simulink model "adaptive_observer_for_sin_signal_original"  (R2021b)
settings: Solver=ode4  StartTime=0.0  StopTime=200.0  FixedStep=0.0001  RelTol=1e-3
model workspace: external: MATLAB File D:\practice\sci\variables2n1.m (data not in the file)
values from neighbouring files (symbols this model uses):
  A = zeros(2*dimension+1 , 2*dimension+1)    [variables2n1.m]
  alpha = [1,3]    [variables2n1.m]
  amp = [1;1]    [variables2n1.m]
  amp_M = [1;1]    [variables2n1.m]
  bias = [0;0]    [variables2n1.m]
  bias_M = [0;0]    [variables2n1.m]
  bigGammaZ0 = zeros(2*dimension+1, dimension)    [variables2n1.m]
  C = zeros(1, 2*dimension+1)    [variables2n1.m]
  delta = C*A    [variables2n1.m]
  dimension = 2    [variables2n1.m]
  freq = [2;3]    [variables2n1.m]
  freq_M = [1.8;3.2]    [variables2n1.m]
  freqSwitcher = 100    [variables2n1.m]
  initialTheta = [initialOmega(1)^2-alpha(1);     initialOmega(2)^2-alpha(2)]    [variables2n1.m]
  initialZ = [1*sin(0); 1*r^2*cos(0)/initialOmega(1);           1*sin(0); 1*r^2*cos(0)/initialOmega(2); 0]    [variables2n1.m]
  L = (place(A',C',eigenvalues))'    [variables2n1.m]
  mu = 2    [variables2n1.m]
  omegaLimiter = sqrt(dimension)*maxOmega    [variables2n1.m]
  phase = [0;0]    [variables2n1.m]
  phase_M = [0;0]    [variables2n1.m]
  r = 1.2    [variables2n1.m]
  turn_mods_on = 0    [variables2n1.m]
  zMax = 5    [variables2n1.m]
undefined symbols (not defined in the file or in its folder): G
settings Model: Creator=ASUS  LastModifiedBy=ASUS

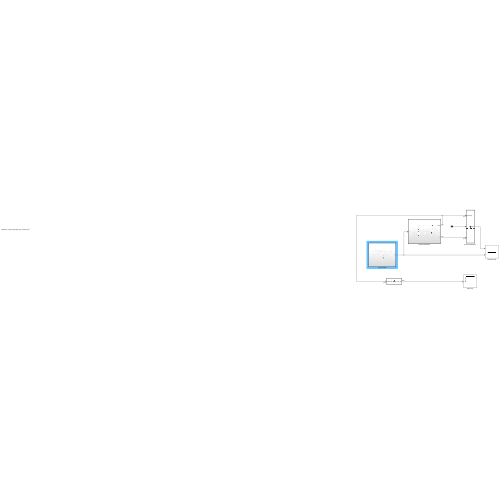
[thumbnail: Simulink's stored preview of the top-level diagram]
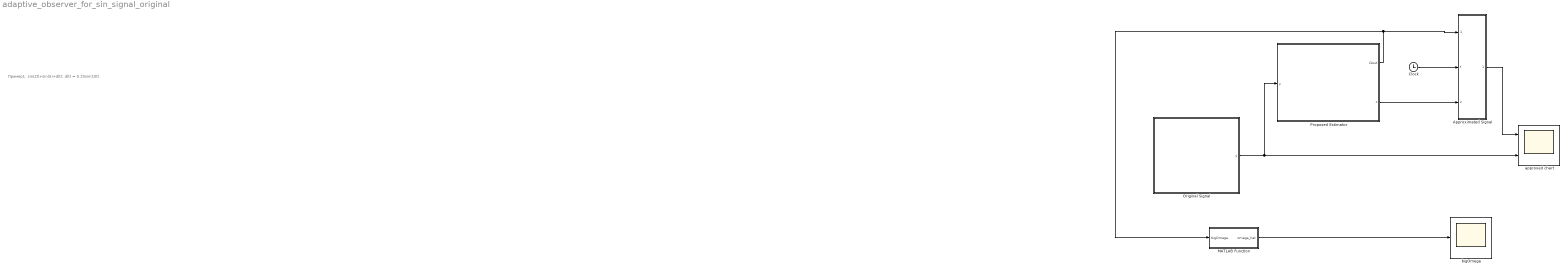
== system adaptive_observer_for_sin_signal_original ==
  note: Пример1. sin(2t)+sin(5)+d(t); d(t) = 0.25sin(10t)
  Approximated Signal : MATLAB Function  TreatAsAtomicUnit=on
  Clock : Clock
  MATLAB Function : MATLAB Function  TreatAsAtomicUnit=on
  Original Signal : Subsystem  Priority=1  TreatAsAtomicUnit=on
  Proposed Estimator : Subsystem  Priority=2  TreatAsAtomicUnit=on
  approxed chart : Scope  NumInputPorts=2
  bigOmega : Scope
  wires:
  Approximated Signal/1(sgn_value) -> approxed chart/1
  Clock/1 -> Approximated Signal/2(t)
  Original Signal/1(y) -> approxed chart/2, Proposed Estimator/1(y)
  Proposed Estimator/2(z) -> Approximated Signal/3(z)
  Proposed Estimator/1(Ωout) -> Approximated Signal/1(bigOmega), MATLAB Function/1(bigOmega)
  MATLAB Function/1(omega_hat) -> bigOmega/1

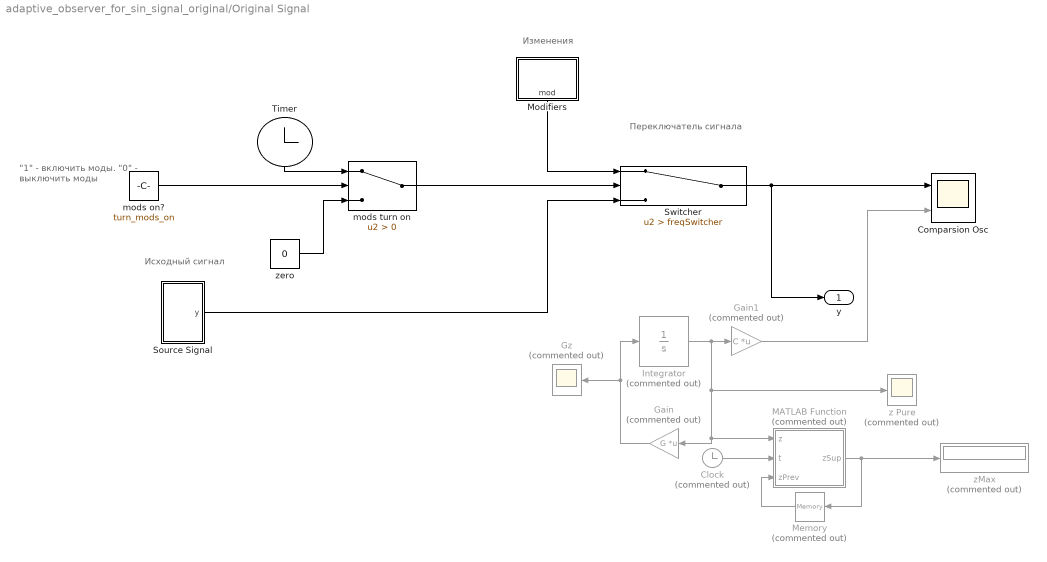
== system adaptive_observer_for_sin_signal_original/Original Signal ==
  note: "1" - включить моды.
      | "0" - выключить моды
  note: Изменения
  note: Переключатель сигнала
  note: Исходный сигнал
  Clock : Clock  Commented=on
  Comparsion Osc : Scope  NumInputPorts=2
  Gain : Gain  Commented=on  Gain=G  Multiplication=Matrix(K*u)
  Gain1 : Gain  Commented=on  Gain=C  Multiplication=Matrix(K*u)
  Gz : Scope  Commented=on
  Integrator : Integrator  Commented=on  InitialCondition=[0;(r^2)/2;0;(r^2)/3;0]
  MATLAB Function : MATLAB Function  Commented=on  TreatAsAtomicUnit=on
  Memory : Memory  Commented=on
  Modifiers : Subsystem
  Source Signal : Subsystem
  Switcher : Switch  Criteria=u2 > Threshold  Threshold=freqSwitcher
  Timer : Clock
  mods on? : Constant  Value=turn_mods_on
  mods turn on : Switch  Criteria=u2 > Threshold
  z Pure : Scope  Commented=on
  zMax : Display  Commented=on
  zero : Constant  Value=0
  y : Outport
  wires:
  Gain/1 -> Gz/1, Integrator/1
  Gain1/1 -> Comparsion Osc/2
  Integrator/1 -> Gain/1, MATLAB Function/1(z), z Pure/1, Gain1/1
  MATLAB Function/1(zSup) -> Memory/1, zMax/1
  Clock/1 -> MATLAB Function/2(t)
  Memory/1 -> MATLAB Function/3(zPrev)
  Source Signal/1(y) -> Switcher/3
  Modifiers/1(mod) -> Switcher/1
  Switcher/1 -> y/1, Comparsion Osc/1
  mods on?/1 -> mods turn on/2
  Timer/1 -> mods turn on/1
  mods turn on/1 -> Switcher/2
  zero/1 -> mods turn on/3

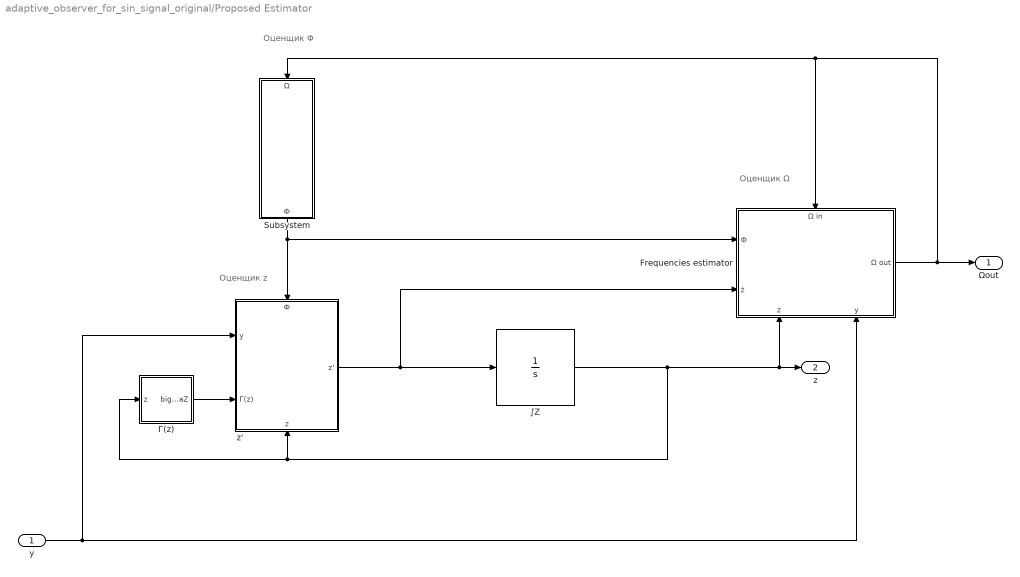
== system adaptive_observer_for_sin_signal_original/Proposed Estimator ==
  note: Оценщик Ω
  note: Оценщик Φ
  note: Оценщик z
  y : Inport
  Frequencies estimator : Subsystem
      settings: PortSchema="{\"entries\":[{\"content\":{\"sides\":[{\"content\":{\"connectorIds\":[\"In1\",\"In2\"]},\"type\":\"ConnectorPlacement.EquallySpacedRectSide\",\"uuid\":\"56415c13-d553-4f88-94d3-75bcdc800e4b\"},{\"content\":{\"connectorIds\":[\"Out1\"],\"side\":\"RIGHT\"},\"type\":\"ConnectorPlacement.EquallySpacedRectSide\",\"uuid\":\"a1bdd2d2-4e49-40cb-b0b7-1df5316e4510\"},{\"content\":{\"connectorIds\":[\"In3\"],\"side\":\"TOP\"},\"type\":\"ConnectorPlacement.EquallySpacedRectSide\",\"uuid\":\"59b6ba3d-4a55-43e8-9b14-0d873cc3c9ca\"},{\"content\":{\"connectorIds\":[\"In4\",\"In5\"],\"side\":\"BOTTOM\"},\"type\":\"ConnectorPlacement.EquallySpacedRectSide\",\"uuid\":\"70a04625-4f15-4458-8acb-2ccaa963f28c\"}]},\"type\":\"ConnectorPlacement.EquallySpacedConnector\",\"uuid\":\"fdf2e112-ecff-41aa-a5cb-d527a9dd51a8\"}],\"packageUris\":[\"http://schema.mathworks.com/mf0/Connector/R2020b\"],\"version\":\"1.0\"}"
  Subsystem : Subsystem  Priority=6  TreatAsAtomicUnit=on
  z' : Subsystem  Priority=7  TreatAsAtomicUnit=on
      settings: PortSchema="{\"entries\":[{\"content\":{\"sides\":[{\"content\":{\"connectorIds\":[\"In1\",\"In2\"]},\"type\":\"ConnectorPlacement.EquallySpacedRectSide\",\"uuid\":\"ef8cffdc-1e6f-42c0-8cb3-bf318ca182f8\"},{\"content\":{\"connectorIds\":[\"Out1\"],\"side\":\"RIGHT\"},\"type\":\"ConnectorPlacement.EquallySpacedRectSide\",\"uuid\":\"a9c7e5b7-281a-47aa-808a-eb2877f3eee0\"},{\"content\":{\"connectorIds\":[\"In3\"],\"side\":\"TOP\"},\"type\":\"ConnectorPlacement.EquallySpacedRectSide\",\"uuid\":\"7bb4f6b5-7deb-4e08-9b2d-b96cfbb2c85e\"},{\"content\":{\"connectorIds\":[\"In4\"],\"side\":\"BOTTOM\"},\"type\":\"ConnectorPlacement.EquallySpacedRectSide\",\"uuid\":\"fa3b2d15-5a15-4cf8-893e-51642802107c\"}]},\"type\":\"ConnectorPlacement.EquallySpacedConnector\",\"uuid\":\"64fccc24-315d-40ff-920f-bd434d551c1a\"}],\"packageUris\":[\"http://schema.mathworks.com/mf0/Connector/R2020b\"],\"version\":\"1.0\"}"
  Г(z) : MATLAB Function  Priority=2  TreatAsAtomicUnit=on
  "∫Z " : Integrator  Priority=1  InitialCondition=initialZ
  Ωout : Outport
  z : Outport  Port=2
  wires:
  z'/1(z') -> Frequencies estimator/2(ż), "∫Z "/1
  Г(z)/1(bigGammaZ) -> z'/2(Г(z))
  "∫Z "/1 -> z/1, Frequencies estimator/4(z), Г(z)/1(z), z'/4(z)
  Frequencies estimator/1(Ω out) -> Subsystem/1(Ω), Frequencies estimator/3(Ω in), Ωout/1
  y/1 -> Frequencies estimator/5(y), z'/1(y)
  Subsystem/1(Ф) -> z'/3(Ф), Frequencies estimator/1(Ф)

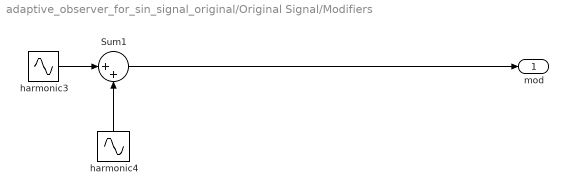
== system adaptive_observer_for_sin_signal_original/Original Signal/Modifiers ==
  Sum1 : Sum  Inputs=|++
  harmonic3 : Sin  Priority=0  Amplitude=amp_M(1)  Bias=bias_M(1)  Frequency=freq_M(1)  Phase=phase_M(1)  SampleTime=0
  harmonic4 : Sin  Priority=0  Amplitude=amp_M(2)  Bias=bias_M(2)  Frequency=freq_M(2)  Phase=phase_M(2)  SampleTime=0
  mod : Outport
  wires:
  harmonic4/1 -> Sum1/2
  harmonic3/1 -> Sum1/1
  Sum1/1 -> mod/1

== system adaptive_observer_for_sin_signal_original/Original Signal/Source Signal ==
  Sum : Sum  Inputs=|++
  harmonic1 : Sin  Priority=0  Amplitude=amp(1)  Bias=bias(1)  Frequency=freq(1)  Phase=phase(1)  SampleTime=0
  harmonic2 : Sin  Priority=0  Amplitude=amp(2)  Bias=bias(2)  Frequency=freq(2)  Phase=phase(2)  SampleTime=0
  y : Outport
  wires:
  harmonic1/1 -> Sum/1
  harmonic2/1 -> Sum/2
  Sum/1 -> y/1

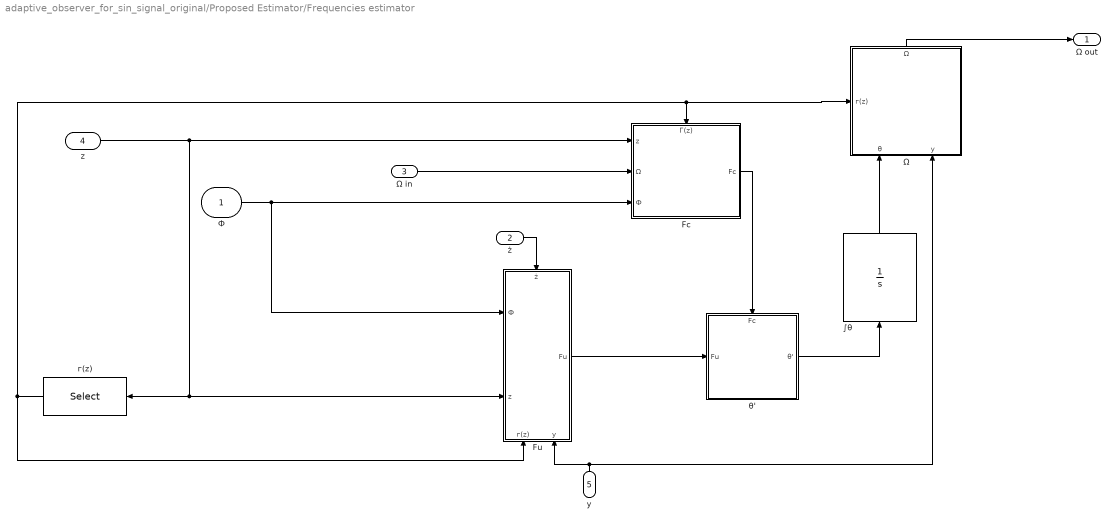
== system adaptive_observer_for_sin_signal_original/Proposed Estimator/Frequencies estimator ==
  Ф : Inport
  ż : Inport  Port=2
  Ω in : Inport  Port=3
  z : Inport  Port=4
  y : Inport  Port=5
  Fc : Subsystem  Priority=8  TreatAsAtomicUnit=on
      settings: PortSchema="{\"entries\":[{\"content\":{\"sides\":[{\"content\":{\"connectorIds\":[\"In1\",\"In2\",\"In3\"]},\"type\":\"ConnectorPlacement.EquallySpacedRectSide\",\"uuid\":\"ef8cffdc-1e6f-42c0-8cb3-bf318ca182f8\"},{\"content\":{\"connectorIds\":[\"Out1\"],\"side\":\"RIGHT\"},\"type\":\"ConnectorPlacement.EquallySpacedRectSide\",\"uuid\":\"a9c7e5b7-281a-47aa-808a-eb2877f3eee0\"},{\"content\":{\"connectorIds\":[\"In4\"],\"side\":\"TOP\"},\"type\":\"ConnectorPlacement.EquallySpacedRectSide\",\"uuid\":\"7bb4f6b5-7deb-4e08-9b2d-b96cfbb2c85e\"},{\"content\":{\"connectorIds\":[],\"side\":\"BOTTOM\"},\"type\":\"ConnectorPlacement.EquallySpacedRectSide\",\"uuid\":\"d628d464-6f95-4c60-8de5-a9188665a8a2\"}]},\"type\":\"ConnectorPlacement.EquallySpacedConnector\",\"uuid\":\"64fccc24-315d-40ff-920f-bd434d551c1a\"}],\"packageUris\":[\"http://schema.mathworks.com/mf0/Connector/R2020b\"],\"version\":\"1.0\"}"
  Fu : Subsystem  Priority=9  TreatAsAtomicUnit=on
      settings: PortSchema="{\"entries\":[{\"content\":{\"sides\":[{\"content\":{\"connectorIds\":[\"In1\",\"In2\"]},\"type\":\"ConnectorPlacement.EquallySpacedRectSide\",\"uuid\":\"56415c13-d553-4f88-94d3-75bcdc800e4b\"},{\"content\":{\"connectorIds\":[\"Out1\"],\"side\":\"RIGHT\"},\"type\":\"ConnectorPlacement.EquallySpacedRectSide\",\"uuid\":\"a1bdd2d2-4e49-40cb-b0b7-1df5316e4510\"},{\"content\":{\"connectorIds\":[\"In3\"],\"side\":\"TOP\"},\"type\":\"ConnectorPlacement.EquallySpacedRectSide\",\"uuid\":\"59b6ba3d-4a55-43e8-9b14-0d873cc3c9ca\"},{\"content\":{\"connectorIds\":[\"In4\",\"In5\"],\"side\":\"BOTTOM\"},\"type\":\"ConnectorPlacement.EquallySpacedRectSide\",\"uuid\":\"cb3db39e-f643-4fe7-a27f-76e86359c78d\"}]},\"type\":\"ConnectorPlacement.EquallySpacedConnector\",\"uuid\":\"fdf2e112-ecff-41aa-a5cb-d527a9dd51a8\"}],\"packageUris\":[\"http://schema.mathworks.com/mf0/Connector/R2020b\"],\"version\":\"1.0\"}"
  Ω : Subsystem  Priority=5  TreatAsAtomicUnit=on
      settings: PortSchema="{\"entries\":[{\"content\":{\"sides\":[{\"content\":{\"connectorIds\":[\"In1\",\"In2\"]},\"type\":\"ConnectorPlacement.EquallySpacedRectSide\",\"uuid\":\"0172ca52-64e8-432c-895c-e5829558e278\"},{\"content\":{\"connectorIds\":[\"Out1\"],\"side\":\"RIGHT\"},\"type\":\"ConnectorPlacement.EquallySpacedRectSide\",\"uuid\":\"c83f4e01-5d94-498a-a9de-b4a302d500ab\"},{\"content\":{\"connectorIds\":[\"In3\"],\"side\":\"TOP\"},\"type\":\"ConnectorPlacement.EquallySpacedRectSide\",\"uuid\":\"3a6496e3-470c-4361-9f8f-cd28e1556398\"}]},\"type\":\"ConnectorPlacement.EquallySpacedConnector\",\"uuid\":\"b738ec8a-20ee-4a0a-8362-4988f331d970\"}],\"packageUris\":[\"http://schema.mathworks.com/mf0/Connector/R2020b\"],\"version\":\"1.0\"}"
  θ' : Subsystem  Priority=10  TreatAsAtomicUnit=on
      settings: PortSchema="{\"entries\":[{\"content\":{\"sides\":[{\"content\":{\"connectorIds\":[\"In1\"]},\"type\":\"ConnectorPlacement.EquallySpacedRectSide\",\"uuid\":\"9184f415-d771-478b-8114-38f854f6aad6\"},{\"content\":{\"connectorIds\":[\"Out1\"],\"side\":\"RIGHT\"},\"type\":\"ConnectorPlacement.EquallySpacedRectSide\",\"uuid\":\"399c2935-e635-4d1c-9ba7-451eea57bae3\"},{\"content\":{\"connectorIds\":[\"In2\"],\"side\":\"TOP\"},\"type\":\"ConnectorPlacement.EquallySpacedRectSide\",\"uuid\":\"bdc6ec05-8dca-4996-ba70-702aa29fd179\"}]},\"type\":\"ConnectorPlacement.EquallySpacedConnector\",\"uuid\":\"fa68c3f3-8285-4ee8-b99d-908dba81143c\"}],\"packageUris\":[\"http://schema.mathworks.com/mf0/Connector/R2020b\"],\"version\":\"1.0\"}"
  г(z) : Selector  InputPortWidth=2*dimension+1  IndexOptions=Index vector (dialog)  Indices=2:2:2*dimension  OutputSizes=1
  "∫θ " : Integrator  Priority=3  InitialCondition=initialTheta
  Ω out : Outport
  wires:
  Ф/1 -> Fu/1(Ф), Fc/3(Ф)
  y/1 -> Ω/2(y), Fu/5(y)
  z/1 -> г(z)/1, Fu/2(z), Fc/1(z)
  г(z)/1 -> Fc/4(Г(z)), Ω/3(г(z)), Fu/4(г(z))
  Ω in/1 -> Fc/2(Ω)
  ż/1 -> Fu/3(ż)
  "∫θ "/1 -> Ω/1(θ)
  Ω/1(Ω) -> Ω out/1
  Fc/1(Fc) -> θ'/2(Fc)
  Fu/1(Fu) -> θ'/1(Fu)
  θ'/1(θ') -> "∫θ "/1

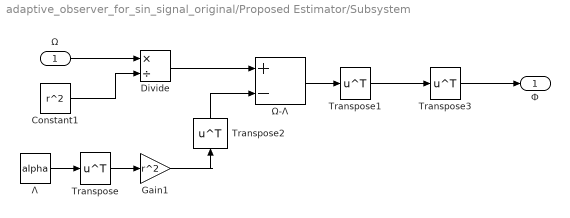
== system adaptive_observer_for_sin_signal_original/Proposed Estimator/Subsystem ==
  Ω : Inport
  Constant1 : Constant  Value=r^2
  Divide : Product  Inputs=*/
  Gain1 : Gain  Gain=r^2
  Transpose{,1..3} (4 alike) : Math  Operator=transpose  SaturateOnIntegerOverflow=on
  Λ : Constant  Value=alpha
  Ω-Λ : Sum  Inputs=+-
  Ф : Outport
  wires:
  Divide/1 -> Ω-Λ/1
  Ω-Λ/1 -> Transpose1/1
  Ω/1 -> Divide/1
  Constant1/1 -> Divide/2
  Gain1/1 -> Transpose2/1
  Λ/1 -> Transpose/1
  Transpose/1 -> Gain1/1
  Transpose2/1 -> Ω-Λ/2
  Transpose1/1 -> Transpose3/1
  Transpose3/1 -> Ф/1

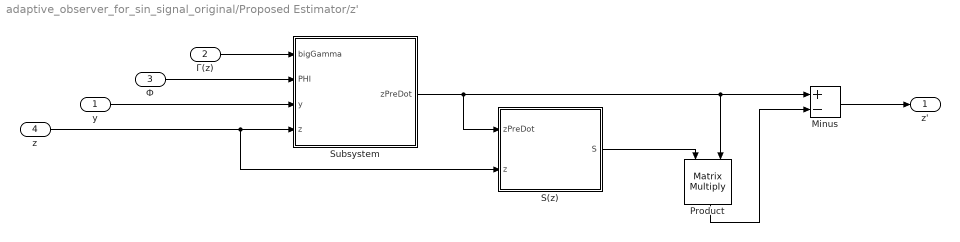
== system adaptive_observer_for_sin_signal_original/Proposed Estimator/z' ==
  y : Inport
  Г(z) : Inport  Port=2
  Ф : Inport  Port=3
  z : Inport  Port=4
  Minus : Sum  Inputs=+-
  Product : Product  Multiplication=Matrix(*)
  S(z) : Subsystem
  Subsystem : Subsystem
  z' : Outport
  wires:
  z/1 -> Subsystem/4(z), S(z)/2(z)
  Minus/1 -> z'/1
  S(z)/1(S) -> Product/1
  Product/1 -> Minus/2
  Subsystem/1(zPreDot) -> Minus/1, Product/2, S(z)/1(zPreDot)
  Г(z)/1 -> Subsystem/1(bigGamma)
  Ф/1 -> Subsystem/2(PHI)
  y/1 -> Subsystem/3(y)

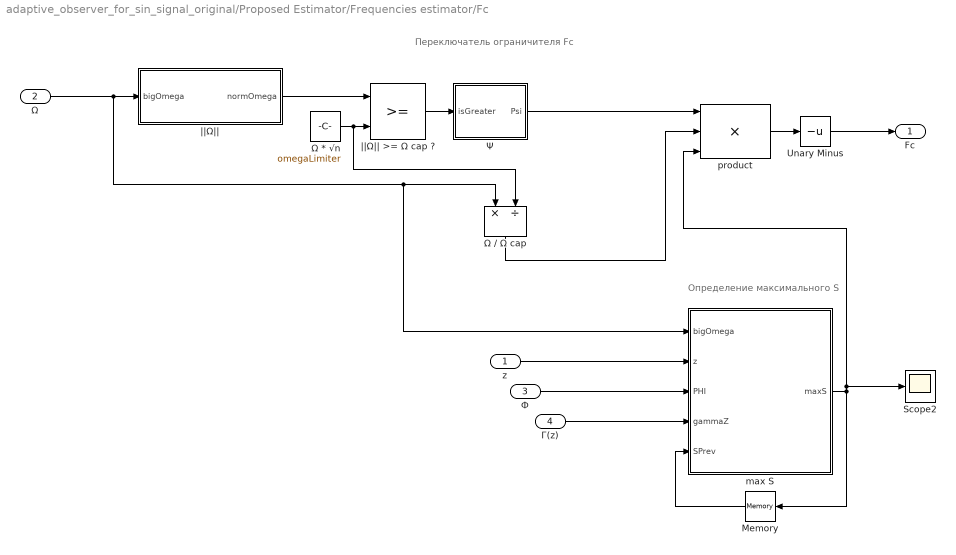
== system adaptive_observer_for_sin_signal_original/Proposed Estimator/Frequencies estimator/Fc ==
  note: Определение максимального S
  note: Переключатель ограничителя Fc
  z : Inport
  Ω : Inport  Port=2
  Ф : Inport  Port=3
  Г(z) : Inport  Port=4
  Memory : Memory
  Scope2 : Scope
  Unary Minus : UnaryMinus
  max S : MATLAB Function  TreatAsAtomicUnit=on
  product : Product  Inputs=3
  ||Ω|| : MATLAB Function  TreatAsAtomicUnit=on
  "||Ω|| >= Ω cap ? " : RelationalOperator  OutDataTypeStr=boolean  RndMeth=Simplest
  Ψ : MATLAB Function  TreatAsAtomicUnit=on
  Ω * √n : Constant  Value=omegaLimiter
  Ω / Ω cap : Product  Inputs=*/
  Fc : Outport
  wires:
  Ф/1 -> max S/3(PHI)
  Ω/1 -> Ω / Ω cap/1, max S/1(bigOmega), ||Ω||/1(bigOmega)
  max S/1(maxS) -> product/3, Scope2/1, Memory/1
  Г(z)/1 -> max S/4(gammaZ)
  z/1 -> max S/2(z)
  ||Ω||/1(normOmega) -> "||Ω|| >= Ω cap ? "/1
  Ω * √n/1 -> Ω / Ω cap/2, "||Ω|| >= Ω cap ? "/2
  "||Ω|| >= Ω cap ? "/1 -> Ψ/1(isGreater)
  Ψ/1(Psi) -> product/1
  Ω / Ω cap/1 -> product/2
  product/1 -> Unary Minus/1
  Unary Minus/1 -> Fc/1
  Memory/1 -> max S/5(SPrev)

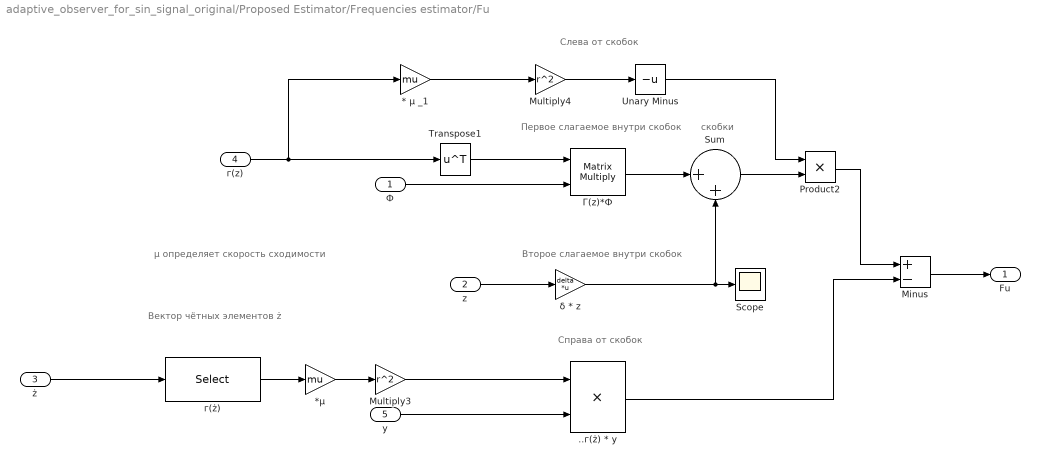
== system adaptive_observer_for_sin_signal_original/Proposed Estimator/Frequencies estimator/Fu ==
  note: Вектор чётных элементов ż
  note: μ определяет скорость сходимости
  note: скобки
  note: Первое слагаемое внутри скобок
  note: Второе слагаемое внутри скобок
  note: Слева от скобок
  note: Справа от скобок
  Ф : Inport
  z : Inport  Port=2
  ż : Inport  Port=3
  г(z) : Inport  Port=4
  y : Inport  Port=5
  * μ _1 : Gain  Gain=mu
  *μ : Gain  Gain=mu
  ..г(ż) * y : Product
  Minus : Sum  Inputs=+-
  Multiply3 : Gain  Gain=r^2
  Multiply4 : Gain  Gain=r^2
  Product2 : Product
  Scope : Scope
  Sum : Sum  Inputs=|++
  Transpose1 : Math  Operator=transpose  SaturateOnIntegerOverflow=on
  Unary Minus : UnaryMinus
  δ * z : Gain  Gain=delta  Multiplication=Matrix(K*u)
  Г(z)*Ф : Product  Multiplication=Matrix(*)
  г(ż) : Selector  InputPortWidth=2*dimension+1  IndexOptions=Index vector (dialog)  Indices=2:2:2*dimension  OutputSizes=1
  Fu : Outport
  wires:
  ż/1 -> г(ż)/1
  г(z)/1 -> * μ _1/1, Transpose1/1
  *μ/1 -> Multiply3/1
  г(ż)/1 -> *μ/1
  Multiply3/1 -> ..г(ż) * y/1
  y/1 -> ..г(ż) * y/2
  Transpose1/1 -> Г(z)*Ф/1
  * μ _1/1 -> Multiply4/1
  Multiply4/1 -> Unary Minus/1
  z/1 -> δ * z/1
  Г(z)*Ф/1 -> Sum/1
  δ * z/1 -> Scope/1, Sum/2
  Unary Minus/1 -> Product2/1
  Sum/1 -> Product2/2
  Product2/1 -> Minus/1
  ..г(ż) * y/1 -> Minus/2
  Minus/1 -> Fu/1
  Ф/1 -> Г(z)*Ф/2

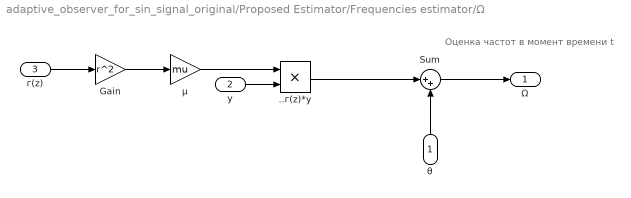
== system adaptive_observer_for_sin_signal_original/Proposed Estimator/Frequencies estimator/Ω ==
  note: Оценка частот в момент времени t
  θ : Inport
  y : Inport  Port=2
  г(z) : Inport  Port=3
  ..г(z)*y : Product
  Gain : Gain  Gain=r^2
  Sum : Sum  Inputs=|++
  μ : Gain  Gain=mu
  Ω : Outport
  wires:
  г(z)/1 -> Gain/1
  Gain/1 -> μ/1
  μ/1 -> ..г(z)*y/1
  y/1 -> ..г(z)*y/2
  ..г(z)*y/1 -> Sum/1
  θ/1 -> Sum/2
  Sum/1 -> Ω/1

== system adaptive_observer_for_sin_signal_original/Proposed Estimator/Frequencies estimator/θ' ==
  note: Образует основу θ'
  note: Удерживает Ω в области определения
  Fu : Inport
  Fc : Inport  Port=2
  Sum : Sum  Inputs=|++
  θ' : Outport
  wires:
  Fu/1 -> Sum/2
  Sum/1 -> θ'/1
  Fc/1 -> Sum/1

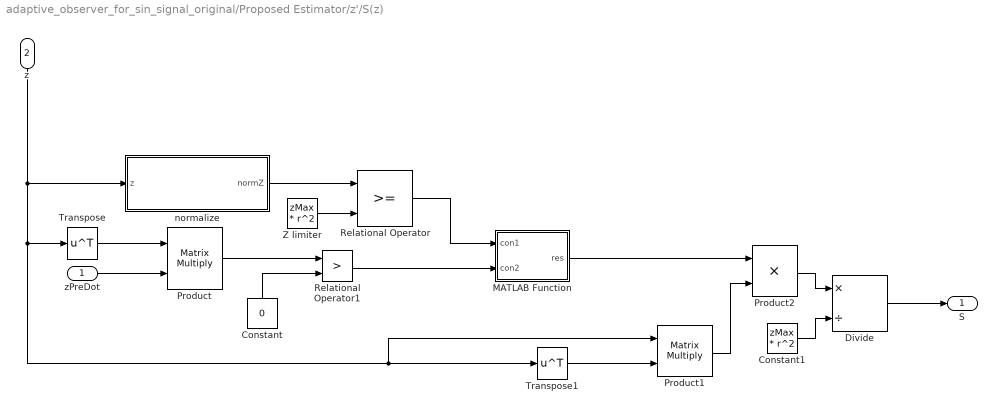
== system adaptive_observer_for_sin_signal_original/Proposed Estimator/z'/S(z) ==
  zPreDot : Inport
  z : Inport  Port=2
  Constant : Constant  Value=0
  Constant1 : Constant  Value=zMax * r^2
  Divide : Product  Inputs=*/
  MATLAB Function : MATLAB Function  TreatAsAtomicUnit=on
  Product : Product  Multiplication=Matrix(*)
  Product1 : Product  Multiplication=Matrix(*)
  Product2 : Product
  Relational Operator : RelationalOperator  OutDataTypeStr=boolean  RndMeth=Simplest
  Relational Operator1 : RelationalOperator  Operator=>  OutDataTypeStr=boolean  RndMeth=Simplest
  Transpose : Math  Operator=transpose  SaturateOnIntegerOverflow=on
  Transpose1 : Math  Operator=transpose  SaturateOnIntegerOverflow=on
  Z limiter : Constant  Value=zMax * r^2
  normalize : MATLAB Function  TreatAsAtomicUnit=on
  S : Outport
  wires:
  Z limiter/1 -> Relational Operator/2
  normalize/1(normZ) -> Relational Operator/1
  Relational Operator/1 -> MATLAB Function/1(con1)
  z/1 -> Product1/1, Transpose1/1, Transpose/1, normalize/1(z)
  Transpose/1 -> Product/1
  zPreDot/1 -> Product/2
  Product/1 -> Relational Operator1/1
  Constant/1 -> Relational Operator1/2
  Relational Operator1/1 -> MATLAB Function/2(con2)
  MATLAB Function/1(res) -> Product2/1
  Transpose1/1 -> Product1/2
  Product1/1 -> Product2/2
  Product2/1 -> Divide/1
  Constant1/1 -> Divide/2
  Divide/1 -> S/1

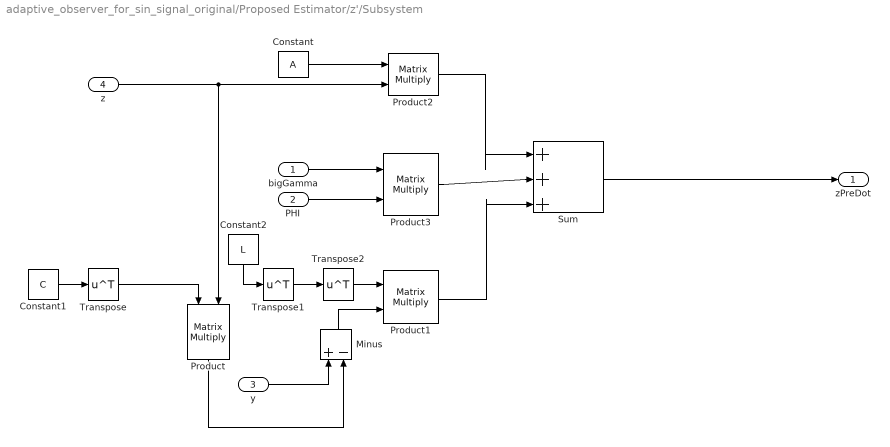
== system adaptive_observer_for_sin_signal_original/Proposed Estimator/z'/Subsystem ==
  bigGamma : Inport
  PHI : Inport  Port=2
  y : Inport  Port=3
  z : Inport  Port=4
  Constant : Constant  Value=A
  Constant1 : Constant  Value=C
  Constant2 : Constant  Value=L
  Minus : Sum  Inputs=+-
  Product{,1..3} (4 alike) : Product  Multiplication=Matrix(*)
  Sum : Sum  Inputs=|+++
  Transpose : Math  Operator=transpose  SaturateOnIntegerOverflow=on
  Transpose1 : Math  Operator=transpose  SaturateOnIntegerOverflow=on
  Transpose2 : Math  Operator=transpose  SaturateOnIntegerOverflow=on
  zPreDot : Outport
  wires:
  z/1 -> Product2/2, Product/2
  Sum/1 -> zPreDot/1
  Constant1/1 -> Transpose/1
  y/1 -> Minus/1
  Product/1 -> Minus/2
  Constant2/1 -> Transpose1/1
  Minus/1 -> Product1/2
  Constant/1 -> Product2/1
  bigGamma/1 -> Product3/1
  PHI/1 -> Product3/2
  Product2/1 -> Sum/1
  Product3/1 -> Sum/2
  Product1/1 -> Sum/3
  Transpose/1 -> Product/1
  Transpose2/1 -> Product1/1
  Transpose1/1 -> Transpose2/1

== matlab function adaptive_observer_for_sin_signal_original/Approximated Signal ==
  data: bigOmega input size=[dimension 1]; t input; r parameter size=1; dimension parameter size=1; z input size=[2*dimension+1 1]; sgn_value output
function sgn_value = sgnl_generated(bigOmega, t, r, dimension, z)

z3 = z(end);
z1 = z(1:2:end-1);
z2 = z(2:2:end);

bias = z3;



frequency = zeros(1, dimension);
amplitude = zeros(1, dimension);
phase = zeros (1, dimension);

sgn_value = bias;

for j=1:dimension
    frequency(j) = sqrt(abs(bigOmega(j)));

    amplitude(j) = sqrt(z1(j).^2 + ((frequency(j).^2/r^4).*z2(j).^2));

    phase(j) = angle((frequency(j)/r^2).*z2(j) + 1i*z1(j)) - mod(frequency(j)*t, 2*pi);
    
    phase(j) = mod(phase(j) + pi, 2*pi) - pi;

    sgn_value = (sgn_value + amplitude(j).*sin(frequency(j)*t + phase(j)));
end

== matlab function adaptive_observer_for_sin_signal_original/Proposed Estimator/z'/S(z)/MATLAB Function ==
  data: con1 input; res output; con2 input
function res = fcn(con1, con2)

if (con1 == true) && (con2 == true)
    res = 1;
else
    res = 0;
end

== matlab function adaptive_observer_for_sin_signal_original/Proposed Estimator/Frequencies estimator/Fc/||Ω|| ==
  data: bigOmega input size=[dimension 1]; normOmega output size=1
function normOmega = norma(bigOmega)

normOmega = norm(bigOmega);

== matlab function adaptive_observer_for_sin_signal_original/Proposed Estimator/Frequencies estimator/Fc/Ψ ==
  data: isGreater input; Psi output
function Psi = PSI(isGreater)

if isGreater
    Psi = 1;
else 
    Psi = 0;
end

== matlab function adaptive_observer_for_sin_signal_original/Proposed Estimator/Г(z) ==
  settings: sampleTime=0.1
  data: z input size=[2*dimension+1 1]; bigGammaZ output size=[2*dimension+1 dimension]; dimension parameter size=1; bigGammaZ0 parameter size=[2*dimension+1 dimension]
function bigGammaZ = gms1(z, dimension, bigGammaZ0)

bigGammaZ = bigGammaZ0;
for i = 1:dimension
    bigGammaZ(2*i - 1,i) = z(2*i);
end

== matlab function adaptive_observer_for_sin_signal_original/Original Signal/MATLAB Function ==
  data: z input; t input; zSup output; zPrev input
function zSup = fcn(z, t, zPrev)



if (t == 0)
    zPrev = norm(z);
end

zSup = max(norm(z),zPrev);

== matlab function adaptive_observer_for_sin_signal_original/Proposed Estimator/z'/S(z)/normalize ==
  data: z input size=[2*dimension+1 1]; normZ output size=1
function normZ = norma(z)

normZ = norm(z);

== matlab function adaptive_observer_for_sin_signal_original/Proposed Estimator/Frequencies estimator/Fc/max S ==
  settings: sampleTime=0.1
  data: bigOmega input size=[dimension 1]; z input size=[2*dimension+1 1]; mu parameter size=1; r parameter size=1; delta parameter size=[1 2*dimension+1]; PHI input size=[dimension 1]; maxS output size=1; gammaZ input size=[dimension 1]; SPrev input size=1; dimension parameter size=1
function maxS = SCounter(bigOmega, z, mu, r, delta, PHI, gammaZ, SPrev, dimension)...

    tempSum = 0;

    z2 = z(2:2:end);

    frequency = zeros(dimension,1);
    for i = 1:dimension
        frequency(i) = sqrt(abs(bigOmega(i))); 
    end

    disturbanceDot = 0;

    for i = 1:dimension
        tempSum = tempSum + frequency(i)^2 * z2(i) + disturbanceDot; %1 
    end

    gammaZ = gammaZ';


    maxS = norm(r^2 * mu * gammaZ * tempSum - r^2 * mu * gammaZ ... 
       * (gammaZ * PHI + delta * z));

%     if SPrev >= maxS
%         maxS = SPrev;
%     elseif SPrev < maxS
%         maxS = maxS*1.1;
%     end
    maxS = maxS*1.1;

end

== matlab function adaptive_observer_for_sin_signal_original/MATLAB Function ==
  data: bigOmega input; omega_hat output
function omega_hat = fcn(bigOmega)

omega_hat = sqrt(abs(bigOmega));
